simulink model "modFM"  (Simulink 10.1)
settings: Solver=VariableStepAuto  StartTime=0.0  StopTime=100  RelTol=1e-3
libraries: commsynccomp2 x2
settings Model: Creator=iba  LastModifiedBy=iba
settings DataIOCC: SaveFormat=Dataset  ReturnWorkspaceOutputs=on
settings OptimizationCC: LifeSpan=auto
settings DebuggingCC: UnderspecifiedInitializationDetection=Simplified  MergeDetectMultiDrivingBlocksExec=error  SFUnexpectedBacktrackingDiag=error  SFNoUnconditionalDefaultTransitionDiag=error  SFExecutionAtInitializationDiag=warning  ArithmeticOperatorsInVariantConditions=error
settings HardwareCC: ProdBitPerPointer=64  ProdBitPerSizeT=64  ProdBitPerPtrDiffT=64  ProdLargestAtomicFloat=Float  ProdIntDivRoundTo=Zero  ProdEndianess=LittleEndian  ProdWordSize=64  ProdHWDeviceType=Intel->x86-64 (Windows64)
settings ModelReferenceCC: PropagateSignalLabelsOutOfModel=on
settings SFSimCC: SimUseLocalCustomCode=on  CustomCodeUndefinedFunction=FilterOut
settings RTWCC: RTWUseLocalCustomCode=on
settings CodeAppCC: StateflowObjectComments=off
settings GRTTargetCC: TargetLangStandard=C99 (ISO)  CombineOutputUpdateFcns=on  GRTInterface=off
settings ConfigComp: CovMetricSettings=dwe  CovHtmlReporting=off  CovSaveCumulativeToWorkspaceVar=off  CovSaveSingleToWorkspaceVar=off  CovExternalEMLEnable=on

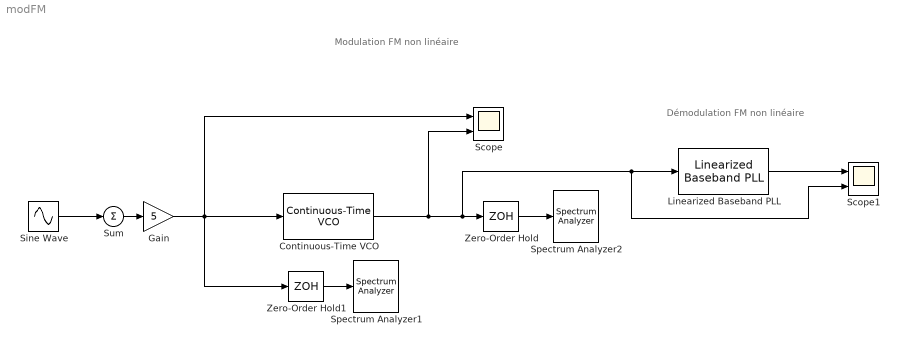
== system modFM ==
  note: Modulation FM non linéaire
  note: Démodulation FM non linéaire
  Continuous-Time VCO : commsynccomp2/Continuous-Time VCO  Ac=1  Fc=25/2/pi  Kc=1  Ph=0
      settings: SourceProductBaseCode=CM
  Gain : Gain  Gain=5
  Linearized Baseband PLL : commsynccomp2/Linearized Baseband PLL  Fn="[3.0002  0  40002]"  Fd="[1   67.46   2270.9   40002]"  Kvco=1
      settings: SourceProductBaseCode=CM
  Scope : Scope  NumInputPorts=2
  Scope1 : Scope  NumInputPorts=2
  Sine Wave : Sin  Amplitude=linspace(0.15,0.1,9)  Frequency=(1:0.5:5)  SampleTime=0
  Spectrum Analyzer1 : SpectrumAnalyzer
  Spectrum Analyzer2 : SpectrumAnalyzer
  Sum : Sum  Inputs=+
  Zero-Order Hold : ZeroOrderHold  SampleTime=0.05
  Zero-Order Hold1 : ZeroOrderHold  SampleTime=0.05
  wires:
  Sine Wave/1 -> Sum/1
  ? -> ?
  Sum/1 -> Gain/1
  Continuous-Time VCO/1 -> Scope/2, Scope1/2, Linearized Baseband PLL/1, Zero-Order Hold/1
  Gain/1 -> Zero-Order Hold1/1, Scope/1, Continuous-Time VCO/1
  Zero-Order Hold1/1 -> Spectrum Analyzer1/1
  Zero-Order Hold/1 -> Spectrum Analyzer2/1
  Linearized Baseband PLL/2 -> Scope1/1
